simulink model "RTDPES_PMS"  (R2026a)
settings: Solver=VariableStepAuto  StopTime=20
libraries: simulink x7, dspsigops x2
settings Model: Creator=chitn  LastModifiedBy=chitn

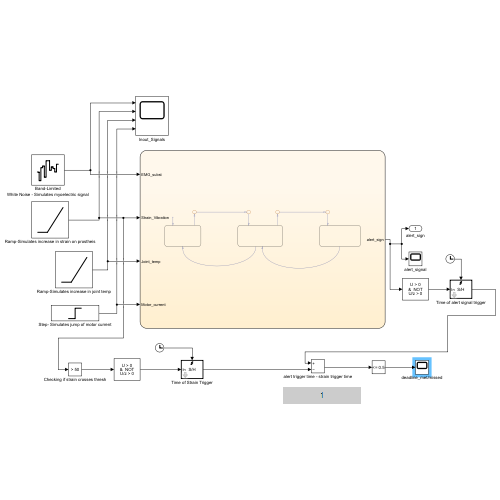
[thumbnail: Simulink's stored preview of the top-level diagram]
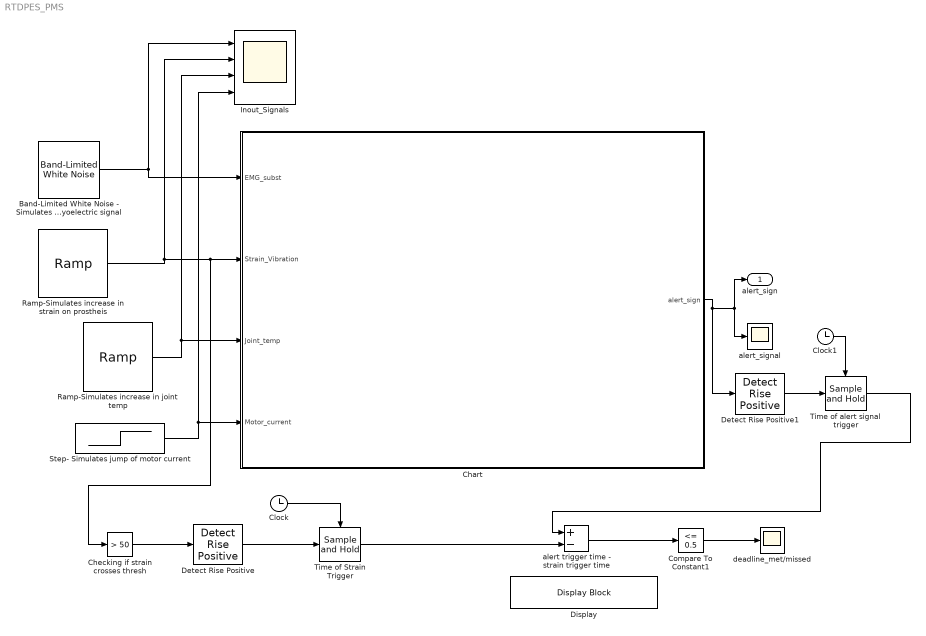
== system RTDPES_PMS ==
  Band-Limited White Noise - Simulates myoelectric signal : simulink/Sources/Band-Limited White Noise  Cov=[0.1]  Ts=0.1  seed=[23341]
  Chart : Stateflow chart  TreatAsAtomicUnit=on
      settings: PortSchema="{\"entries\":[{\"content\":{\"sides\":[{\"content\":{\"connectorIds\":[\"In1\",\"In2\",\"In4\",\"In3\"]},\"type\":\"ConnectorPlacement.EquallySpacedRectSide\",\"uuid\":\"9873ac12-fb94-4960-bf90-b711241cac84\"},{\"content\":{\"connectorIds\":[\"Out1\"],\"side\":\"RIGHT\"},\"type\":\"ConnectorPlacement.EquallySpacedRectSide\",\"uuid\":\"f00dccd1-94c5-487e-9a42-9e2de118c1cb\"},{\"content\":{\"side\":\"TOP\"},\"type\":\"ConnectorPlacement.EquallySpacedRectSide\",\"uuid\":\"20f63af7-62b9-4bcb-83e4-62ffa323d08f\"}]},\"type\":\"ConnectorPlacement.EquallySpacedConnector\",\"uuid\":\"f248f9da-0d82-47bc-ad78-40a795bfe07b\"}],\"packageUris\":[\"http://schema.mathworks.com/mf0/Connector/R2020b\"],\"version\":\"1.0\"}"
  Checking if strain crosses thresh : simulink/Logic and Bit Operations/Compare To Constant  relop=>  const=50  OutDataTypeStr=boolean
  Clock : Clock
  Clock1 : Clock
  Compare To Constant1 : simulink/Logic and Bit Operations/Compare To Constant  relop=<=  const=0.5  OutDataTypeStr=boolean
  Detect Rise Positive : simulink/Logic and Bit Operations/Detect Rise Positive  vinit=0  OutDataTypeStr=boolean
  Detect Rise Positive1 : simulink/Logic and Bit Operations/Detect Rise Positive  vinit=0  OutDataTypeStr=boolean
  Display : DisplayBlock  LabelPosition=Hide  Transparency=1  GridColor=[0.502, 0.502, 0.502]
  Inout_Signals : Scope  NumInputPorts=4
      settings: ActiveDisplayYMinimum=-15.195716729009565  ActiveDisplayYMaximum=112.79952408100107
  Ramp-Simulates increase in joint temp : simulink/Sources/Ramp  slope=4.5  start=0  InitialOutput=0
  Ramp-Simulates increase in strain on prostheis : simulink/Sources/Ramp  slope=5  start=0  InitialOutput=0
  Step- Simulates jump of motor current : Step  Time=2  FinalValue=100  SampleTime=0
  Time of Strain Trigger : dspsigops/Sample and Hold  trig=Rising edge  initCond=0  latchinput=off
  Time of alert signal trigger : dspsigops/Sample and Hold  trig=Rising edge  initCond=0  latchinput=off
  alert trigger time - strain trigger time : Sum  Inputs=+-  OutDataTypeStr=double
  alert_signal : Scope
      settings: ActiveDisplayYMinimum=-16.266653310496466  ActiveDisplayYMaximum=51.118548345239304  YLabel=ALERT TRIGGER STATUS  DataLoggingVariableName=ScopeData2
  deadline_met/missed : Scope
      settings: ActiveDisplayYMinimum=-16.266653310496466  ActiveDisplayYMaximum=51.118548345239304  YLabel=ALERT TRIGGER STATUS
  alert_sign : Outport
  wires:
  Band-Limited White Noise - Simulates myoelectric signal/1 -> Chart/1(EMG_subst), Inout_Signals/1
  Ramp-Simulates increase in strain on prostheis/1 -> Inout_Signals/2, Checking if strain crosses thresh/1, Chart/2(Strain_Vibration)
  Ramp-Simulates increase in joint temp/1 -> Chart/4(Joint_temp), Inout_Signals/3
  Step- Simulates jump of motor current/1 -> Inout_Signals/4, Chart/3(Motor_current)
  Chart/1(alert_sign) -> Detect Rise Positive1/1, alert_signal/1, alert_sign/1
  Clock/1 -> Time of Strain Trigger/Trigger
  Checking if strain crosses thresh/1 -> Detect Rise Positive/1
  Detect Rise Positive/1 -> Time of Strain Trigger/1
  Clock1/1 -> Time of alert signal trigger/Trigger
  Detect Rise Positive1/1 -> Time of alert signal trigger/1
  Time of alert signal trigger/1 -> alert trigger time - strain trigger time/1
  Time of Strain Trigger/1 -> alert trigger time - strain trigger time/2
  alert trigger time - strain trigger time/1 -> Compare To Constant1/1
  Compare To Constant1/1 -> deadline_met/missed/1

== stateflow chart RTDPES_PMS/Chart ==
  state NORMAL
    entry:
    alert_sign = 0;
  state WARNING
  state CRITICAL
    entry:
    alert_sign=1;
  (junction 18) -> (junction 20) : [Strain_Vibration > 50 || Motor_current > 90]
  (junction 25) -> (junction 27) : [Strain_Vibration>80 || Motor_current >90]
  NORMAL -> (junction 18)
  (junction 20) -> WARNING
  WARNING -> (junction 25) [order 1]
  (junction 27) -> CRITICAL
  (default) -> NORMAL
  WARNING -> NORMAL [order 2] : [Strain_Vibration < 50 && Motor_current < 90]
  CRITICAL -> WARNING : [Strain_Vibration < 70 && Motor_current < 90]
  data: EMG_subst input; Strain_Vibration input; Motor_current input; Joint_temp input; alert_sign output
